simulink model "simquat"  (Simulink 6.0)
settings: Solver=ode1  SolverMode=SingleTasking  StartTime=0.0  StopTime=999999  FixedStep=1  MaxStep=1  RelTol=1e-3  AbsTol=1e-6
PostLoadFcn:
  | quatdemo Static Foo Bar
CloseFcn:
  | quatdemo Close
settings Model: Creator=The MathWorks Inc.  LastModifiedBy=batserve  ExtModeAutoUpdateStatusClock=off
settings SolverCC: InitialStep=.1
settings DataIOCC: LimitDataPoints=off  SaveOutput=off  SaveTime=off
settings OptimizationCC: BooleanDataType=off
settings DebuggingCC: CheckExecutionContextPreStartOutputMsg=on  CheckExecutionContextRuntimeOutputMsg=on  SolverPrmCheckMsg=none
settings HardwareCC: TargetUnknown=on

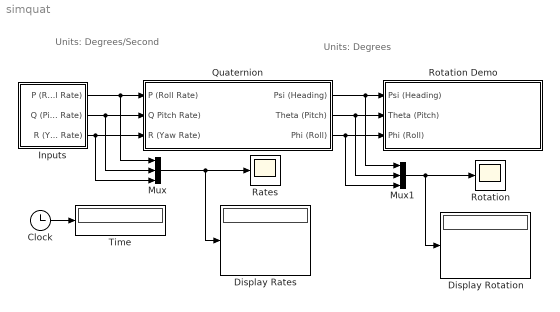
== system simquat ==
  note: Units:
      | Degrees
  note: Units:
      | Degrees/Second
  Clock : Clock
      settings: Decimation=10
  Display Rates : Display
  Display Rotation : Display
  Inputs : Subsystem  PropExecContextAcrossSSBoundary=on
      settings: OpenFcn=quatdemo Dynamic Foo Bar
  Mux : Mux  Inputs=3
  Mux1 : Mux  Inputs=3
  Quaternion : Subsystem  PropExecContextAcrossSSBoundary=on  mask(Quaternion Calculation){Psi=0, Theta=0, Phi=0}
      mask prompts: Psi "Initial Psi Value (Deg.)"; Theta "Initial Theta Value (Deg.):"; Phi "Initial Phi Value (Deg.):"
      mask help: Calculate Psi, Theta and Phi based on P,Q,R
      settings: OpenFcn=quatdemo Static Foo Bar
      mask Help: This block calculates the Yaw (Psi), Pitch (Theta) and Roll (Phi) of an aircraft using quaternion rotation calculations.  The inputs to the block are P (Roll rate), Q(Pitch rate) and R(Yaw rate).  All input units are Degrees per second.  The outputs of the block are Psi, Theta and Phi all given in Degrees.
      mask Display: disp('Quaternion\nCalculation')
  Rates : Scope
      settings: TickLabels=on  DataFormat=Array
  Rotation : Scope
      settings: TickLabels=on  DataFormat=Array
  Rotation Demo : Subsystem  PropExecContextAcrossSSBoundary=on
      settings: OpenFcn=quatdemo Static Foo Bar
      mask Type: Euler Rotation
      mask Display: disp('Euler\nRotation')
  Time : Display
  wires:
  Clock/1 -> Time/1
  Mux1/1 -> Display Rotation/1, Rotation/1
  Quaternion/3(Phi (Roll)) -> Mux1/3, Rotation Demo/3(Phi (Roll))
  Quaternion/2(Theta (Pitch)) -> Mux1/2, Rotation Demo/2(Theta (Pitch))
  Quaternion/1(Psi (Heading)) -> Mux1/1, Rotation Demo/1(Psi (Heading))
  Inputs/3(R (Yaw Rate)) -> Mux/3, Quaternion/3(R (Yaw Rate))
  Inputs/2(Q (Pitch Rate)) -> Mux/2, Quaternion/2(Q Pitch Rate))
  Inputs/1(P (Roll Rate)) -> Mux/1, Quaternion/1(P (Roll Rate))
  Mux/1 -> Rates/1, Display Rates/1

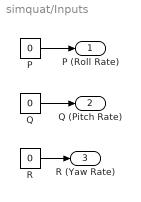
== system simquat/Inputs ==
  P : Constant  Value=0
  Q : Constant  Value=0
  R : Constant  Value=0
  P (Roll Rate) : Outport  InitialOutput=0
  Q (Pitch Rate) : Outport  Port=2  InitialOutput=0
  R (Yaw Rate) : Outport  Port=3  InitialOutput=0
  wires:
  R/1 -> R (Yaw Rate)/1
  Q/1 -> Q (Pitch Rate)/1
  P/1 -> P (Roll Rate)/1

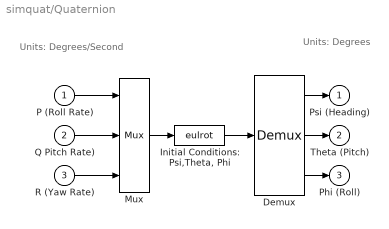
== system simquat/Quaternion ==
  note: Units:
      | Degrees
  note: Units:
      | Degrees/Second
  P (Roll Rate) : Inport  Port=1  LatchInput=off
  Q Pitch Rate) : Inport  Port=2  LatchInput=off
  R (Yaw Rate) : Inport  Port=3  LatchInput=off
  Demux : Demux  Outputs=3
  "Initial Conditions: Psi,Theta, Phi" : S-Function  FunctionName=eulrot  Parameters=Psi,Theta,Phi
  Mux : Mux  Inputs=3
  Psi (Heading) : Outport  InitialOutput=0
  Theta (Pitch) : Outport  Port=2  InitialOutput=0
  Phi (Roll) : Outport  Port=3  InitialOutput=0
  wires:
  Demux/3 -> Phi (Roll)/1
  Demux/2 -> Theta (Pitch)/1
  Demux/1 -> Psi (Heading)/1
  "Initial Conditions: Psi,Theta, Phi"/1 -> Demux/1
  R (Yaw Rate)/1 -> Mux/3
  Q Pitch Rate)/1 -> Mux/2
  P (Roll Rate)/1 -> Mux/1
  Mux/1 -> "Initial Conditions: Psi,Theta, Phi"/1

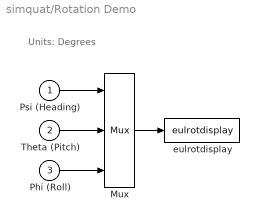
== system simquat/Rotation Demo ==
  note: Units:
      | Degrees
  Psi (Heading) : Inport  Port=1  LatchInput=off
  Theta (Pitch) : Inport  Port=2  LatchInput=off
  Phi (Roll) : Inport  Port=3  LatchInput=off
  Mux : Mux  Inputs=3
  eulrotdisplay : S-Function  FunctionName=eulrotdisplay
  wires:
  Phi (Roll)/1 -> Mux/3
  Theta (Pitch)/1 -> Mux/2
  Psi (Heading)/1 -> Mux/1
  Mux/1 -> eulrotdisplay/1
